simulink model "simulation_GyrosModel"  (R2023b)
settings: Solver=VariableStepAuto  StartTime=0.0  StopTime=10.0  RelTol=1e-3
values from neighbouring files (symbols this model uses):
  i_dConfigMat_IMUfromSCB = eye(3)    [main_GyrosModel.m]
  i_dOrthogErrMatrix = eye(3)    [main_GyrosModel.m]
  i_dScaleFactor = ones(3, 1)    [main_GyrosModel.m]
  i_dSigmaARW = 1E-5    (= 1e-05)    [main_GyrosModel.m]
  i_dSigmaRRW = 0.001    [main_GyrosModel.m]
settings Model: Creator=peterc  LastModifiedBy=peterc

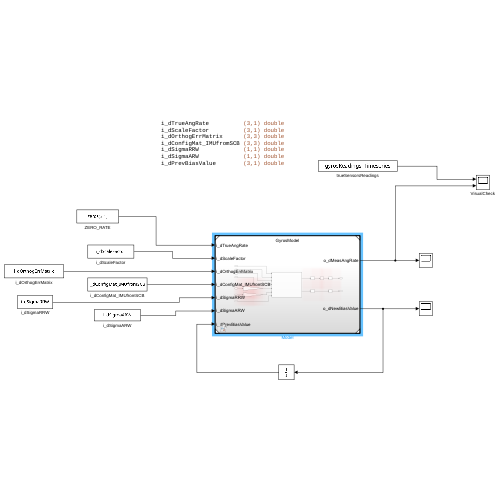
[thumbnail: Simulink's stored preview of the top-level diagram]
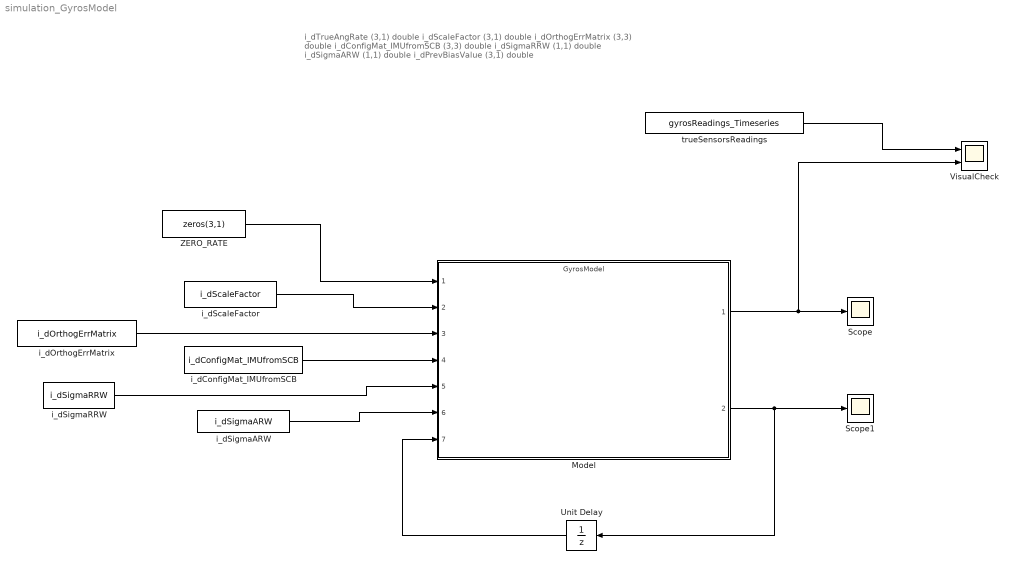
== system simulation_GyrosModel ==
  note: i_dTrueAngRate (3,1) double
      | i_dScaleFactor (3,1) double
      | i_dOrthogErrMatrix (3,3) double
      | i_dConfigMat_IMUfromSCB (3,3) double
      | i_dSigmaRRW (1,1) double
      | i_dSigmaARW (1,1) double
      | i_dPrevBiasValue (3,1) double
  Model : ModelReference  ModelNameDialog=GyrosModel.slx  SimulationMode=Normal  ModelReferenceVersion=1.12
  Scope : Scope
  Scope1 : Scope
  Unit Delay : UnitDelay  SampleTime=-1  HasFrameUpgradeWarning=on
  VisualCheck : Scope  NumInputPorts=2
  ZERO_RATE : Constant  Value=zeros(3,1)  OutDataTypeStr=double
  i_dConfigMat_IMUfromSCB : Constant  Value=i_dConfigMat_IMUfromSCB
  i_dOrthogErrMatrix : Constant  Value=i_dOrthogErrMatrix
  i_dScaleFactor : Constant  Value=i_dScaleFactor
  i_dSigmaARW : Constant  Value=i_dSigmaARW
  i_dSigmaRRW : Constant  Value=i_dSigmaRRW
  trueSensorsReadings : FromWorkspace  VariableName=gyrosReadings_Timeseries  SampleTime=-1  OutputAfterFinalValue=Setting to zero
  wires:
  Model/1 -> VisualCheck/2, Scope/1
  Model/2 -> Unit Delay/1, Scope1/1
  Unit Delay/1 -> Model/7
  i_dSigmaRRW/1 -> Model/5
  i_dSigmaARW/1 -> Model/6
  i_dConfigMat_IMUfromSCB/1 -> Model/4
  i_dOrthogErrMatrix/1 -> Model/3
  i_dScaleFactor/1 -> Model/2
  ZERO_RATE/1 -> Model/1
  trueSensorsReadings/1 -> VisualCheck/1
